simulink model "Segwaysin"  (Simulink 8.2)
settings: Solver=ode45  StartTime=0.0  StopTime=20  MaxStep=1  RelTol=1e-8
settings Model: Creator=La  LastModifiedBy=La

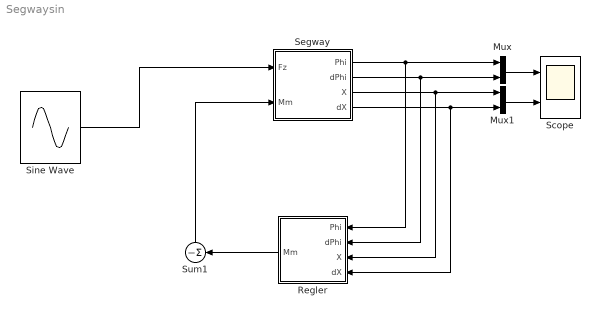
== system Segwaysin ==
  Mux : Mux  Inputs=2
  Mux1 : Mux  Inputs=2
  Regler : Subsystem
  Scope : Scope  NumInputPorts=2
      settings: YMin=-5~-5  YMax=5~5
  Segway : Subsystem
  Sine Wave : Sin  SampleTime=0
  Sum1 : Sum  Inputs=|-
  wires:
  Segway/1(Phi) -> Mux/1, Regler/1(Phi)
  Segway/2(dPhi) -> Mux/2, Regler/2(dPhi)
  Segway/3(X) -> Mux1/1, Regler/3(X)
  Segway/4(dX) -> Mux1/2, Regler/4(dX)
  Mux/1 -> Scope/1
  Mux1/1 -> Scope/2
  Regler/1(Mm) -> Sum1/1
  Sum1/1 -> Segway/2(Mm)
  Sine Wave/1 -> Segway/1(Fz)

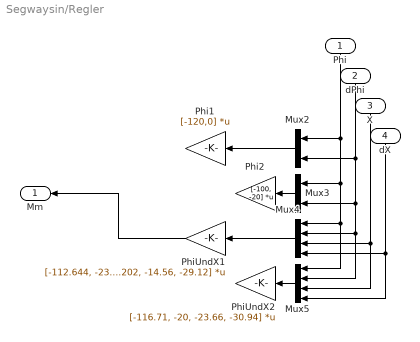
== system Segwaysin/Regler ==
  Phi : Inport
  dPhi : Inport  Port=2
  X : Inport  Port=3
  dX : Inport  Port=4
  Mux2 : Mux  Inputs=2
  Mux3 : Mux  Inputs=2
  Mux4 : Mux
  Mux5 : Mux
  Phi1 : Gain  Gain=[-120,0]  Multiplication=Matrix(K*u)
  Phi2 : Gain  Gain=[-100, -20]  Multiplication=Matrix(K*u)
  PhiUndX1 : Gain  Gain=[-112.644, -23.202, -14.56, -29.12]  Multiplication=Matrix(K*u)
  PhiUndX2 : Gain  Gain=[-116.71, -20, -23.66, -30.94]  Multiplication=Matrix(K*u)
  Mm : Outport
  wires:
  PhiUndX1/1 -> Mm/1
  Mux2/1 -> Phi1/1
  Mux3/1 -> Phi2/1
  Mux4/1 -> PhiUndX1/1
  Mux5/1 -> PhiUndX2/1
  Phi/1 -> Mux2/1, Mux3/1, Mux4/1, Mux5/1
  dPhi/1 -> Mux2/2, Mux3/2, Mux4/2, Mux5/2
  X/1 -> Mux4/3, Mux5/3
  dX/1 -> Mux4/4, Mux5/4

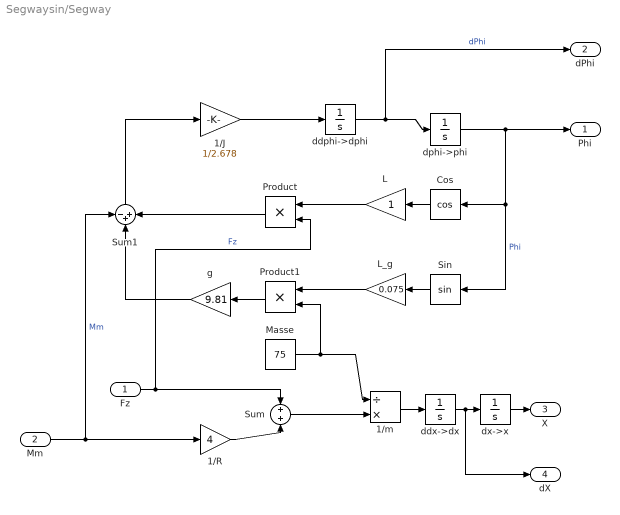
== system Segwaysin/Segway ==
  Fz : Inport
  Mm : Inport  Port=2
  1/J : Gain  Gain=1/2.678
  1/R : Gain  Gain=4
  1/m : Product  Inputs=/*
  Cos : Trigonometry  Operator=cos
  L : Gain
  L_g : Gain  Gain=0.075
  Masse : Constant  Value=75
  Product : Product  RndMeth=Zero
  Product1 : Product  RndMeth=Zero
  Sin : Trigonometry
  Sum : Sum  Inputs=+|+
  Sum1 : Sum  Inputs=-++
  ddphi->dphi : Integrator
  ddx->dx : Integrator
  dphi->phi : Integrator  InitialCondition=0.1
  dx->x : Integrator
  g : Gain  Gain=9.81
  Phi : Outport
  dPhi : Outport  Port=2
  X : Outport  Port=3
  dX : Outport  Port=4
  wires:
  L/1 -> Product/1
  Cos/1 -> L/1
  Sin/1 -> L_g/1
  Product1/1 -> g/1
  dphi->phi/1 -> Phi/1, Cos/1, Sin/1  "Phi"
  1/m/1 -> ddx->dx/1
  ddphi->dphi/1 -> dphi->phi/1, dPhi/1  "dPhi"
  1/J/1 -> ddphi->dphi/1
  ddx->dx/1 -> dx->x/1, dX/1
  dx->x/1 -> X/1
  L_g/1 -> Product1/1
  Masse/1 -> Product1/2, 1/m/1
  Mm/1 -> 1/R/1, Sum1/1  "Mm"
  Sum/1 -> 1/m/2
  1/R/1 -> Sum/2
  Fz/1 -> Sum/1, Product/2  "Fz"
  Product/1 -> Sum1/3
  Sum1/1 -> 1/J/1
  g/1 -> Sum1/2
